simulink model "Aircraft_Simple_Fdm"  (R2022b)
settings: Solver=VariableStepAuto  StartTime=0.0  StopTime=10.0  RelTol=1e-3
libraries: aerolibactuator x4, aerolibv1 x1, uavalgslib x1, aerolibanimutils x1, aerolibpropulsion2 x1
settings Model: Creator=angga  LastModifiedBy=angga

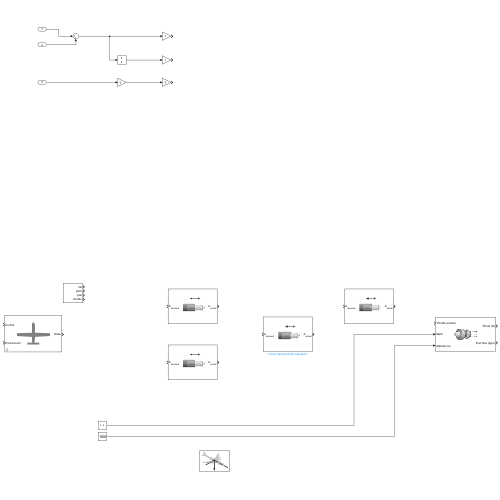
[thumbnail: Simulink's stored preview of the top-level diagram]
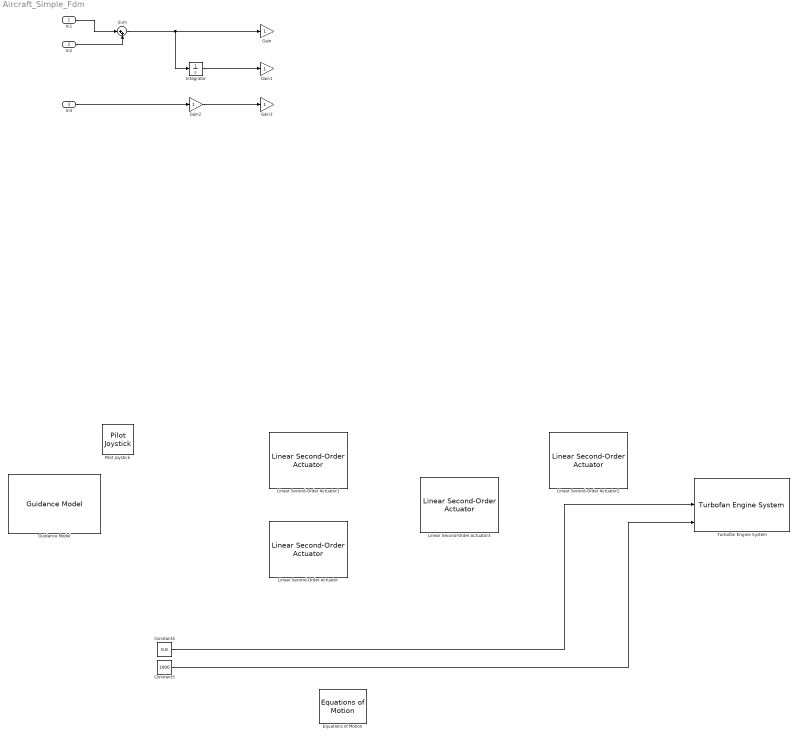
== system Aircraft_Simple_Fdm ==
  In1 : Inport
  In2 : Inport  Port=2
  In3 : Inport  Port=3
  Constant4 : Constant  Value=0.8
  Constant5 : Constant  Value=1000
  Equations of Motion : aerolibv1/Equations of Motion  SystemSampleTime=-1  VariantActivationTime=update diagram  Latency=0  AutoFrameSizeCalculation=off
  Gain{,1..3} (4 alike) : Gain
  Guidance Model : uavalgslib/Guidance Model  ModelType=FixedWingGuidance  SpecifiedDataType=double  SimulateUsing=Code generation  InitialWorldPositionMultirotor=[0; 0; 0]  InitialWorldVelocityMultirotor=[0; 0; 0]  InitialEulerZYXMultirotor=[0; 0; 0]  InitialBodyAngularRateRPYMultirotor=[0; 0; 0]  InitialThrustMultirotor=0  InitialNorthFixedWing=0  InitialEastFixedWing=0  InitialHeightFixedWing=0  InitialAirSpeedFixedWing=0  InitialHeadingAngleFixedWing=0  InitialFlightPathAngleFixedWing=0  InitialRollAngleFixedWing=0  InitialRollAngleRateFixedWing=0  PDRollMultirotor=[3402.97,116.67]  PDPitchMultirotor=[3402.97, 116.67]  PYawRateMultirotor=1950  PThrustMultirotor=3900  MassMultirotor=0.1  PHeightFixedWing=3.9  PHeadingAngleFixedWing=3.9  PFlightPathAngleFixedWing=39  PDRollFixedWing=[3402.97, 116.67]  PAirSpeedFixedWing=1  FlightPathAngleLimitsFixedWing=[-pi/2, pi/2]  StateBusName='FixedWingGuidanceStateBus'  ControlBusName='FixedWingGuidanceControlBus'  EnvironmentBusName='FixedWingGuidanceEnvironmentBus'  DataType=double
  Integrator : Integrator
  Linear Second-Order Actuator{,1..3} (4 alike) : aerolibactuator/Linear Second-Order Actuator  wn_fin=1  z_fin=0.3  fin_act_0=0  fin_act_vel=0
  Pilot Joystick : aerolibanimutils/Pilot Joystick  JoystickID=Joystick1  OutputConfiguration=FourAxis  SampleTime=1/30
  Sum : Sum  Inputs=|++
  Turbofan Engine System : aerolibpropulsion2/Turbofan Engine System  units=Metric (MKS)  ic_source=Internal  IC=100  Fmax=45000  tau=1  SFC=0.35  Nt=0.9
  wires:
  In1/1 -> Sum/1
  In2/1 -> Sum/2
  Sum/1 -> Integrator/1, Gain/1
  Integrator/1 -> Gain1/1
  In3/1 -> Gain2/1
  Gain2/1 -> Gain3/1
  Constant4/1 -> Turbofan Engine System/2
  Constant5/1 -> Turbofan Engine System/3
